simulink model "example1"  (Simulink 6.5)
settings: Solver=ode45  StartTime=0.0  StopTime=2  RelTol=1e-3
settings Model: Creator=2414589  LastModifiedBy=2414589
settings DebuggingCC: MultiTaskDSMMsg=warning  MultiTaskCondExecSysMsg=none  StrictBusMsg=None
settings RTWCC: IncludeERTFirstTime=on

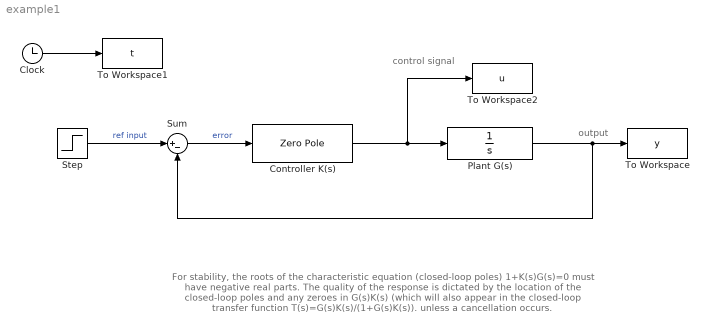
== system example1 ==
  note: control signal
  note: output
  note: For stability, the roots of the characteristic equation (closed-loop poles)
      |
      | 1+K(s)G(s)=0
      |
      | must have negative real parts.  The quality of the response is dictated by the
      | location of the closed-loop poles and any zeroes in G(s)K(s) (which will also
      |  appear in the closed-loop transfer function T(s)=G(s)K(s)/(1+G(s)K(s)).
      |  unless a cancellation occurs.
  Clock : Clock
      settings: Decimation=10
  Controller K(s) : ZeroPole  Poles=[-2 -1]
  Plant G(s) : TransferFcn  Denominator=[1 0]
  Step : Step  Time=0  SampleTime=0
  Sum : Sum  Inputs=|+-
  To Workspace : ToWorkspace  VariableName=y  SampleTime=-1  SaveFormat=Array
  To Workspace1 : ToWorkspace  VariableName=t  SampleTime=-1  SaveFormat=Array
  To Workspace2 : ToWorkspace  VariableName=u  SampleTime=-1  SaveFormat=Array
  wires:
  Step/1 -> Sum/1  "ref input"
  Sum/1 -> Controller K(s)/1  "error"
  Controller K(s)/1 -> To Workspace2/1, Plant G(s)/1
  Plant G(s)/1 -> Sum/2, To Workspace/1
  Clock/1 -> To Workspace1/1
